simulink model "readProximity_sol"  (R2024a)
settings: Solver=FixedStepAuto  StartTime=0.0  StopTime=inf  RelTol=1e-9  EnableMultiTasking=on
undefined symbols (not defined in the file or in its folder): ln
libraries: arduinolib x2
settings Model: ExtModeTrigDuration=2  Creator=twallema  LastModifiedBy=twallema
settings SolverCC: AlgebraicLoopSolver=TrustRegion
settings OptimizationCC: EnhancedBackFolding=on  PassReuseOutputArgsThreshold=0  MaxStackSize=64  OptimizeBlockOrder=speed  DifferentSizesBufferReuse=on  OptimizationCustomize=off
settings DebuggingCC: ParameterTunabilityLossMsg=error  UnconnectedInputMsg=warning  UnconnectedOutputMsg=warning  UnconnectedLineMsg=warning
settings HardwareCC: ProdBitPerInt=16  ProdBitPerPointer=16  ProdBitPerSizeT=16  ProdBitPerPtrDiffT=16  ProdLargestAtomicFloat=None  ProdWordSize=8  ProdHWDeviceType=Atmel->AVR  UseEmbeddedCoderFeatures=off  UseSimulinkCoderFeatures=off
settings ModelReferenceCC: EnableRefExpFcnMdlSchedulingChecks=on
settings SFSimCC: MATLABDynamicMemAlloc=off  CustomCodeUndefinedFunction=UseInterfaceOnly
settings RTWCC: Description=Embedded Coder  SystemTargetFile=ert.tlc  HardwareBoard=Arduino Uno  TemplateMakefile=ert_default_tmf  GenerateReport=on  Toolchain=Arduino AVR  BuildConfiguration=Faster Runs  LaunchReport=on  GPUComputeCapability=3.5  DLArmComputeVersion=19.05
settings CodeAppCC: ForceParamTrailComments=on  OperatorAnnotations=on
settings ERTTargetCC: ERTCustomFileBanners=off  SupportContinuousTime=on  SupportNonInlinedSFcns=on  RemoveResetFunc=off  SupportVariableSizeSignals=on  ModelStepFunctionPrototypeControlCompliant=off  ExtModeStaticAllocSize=250

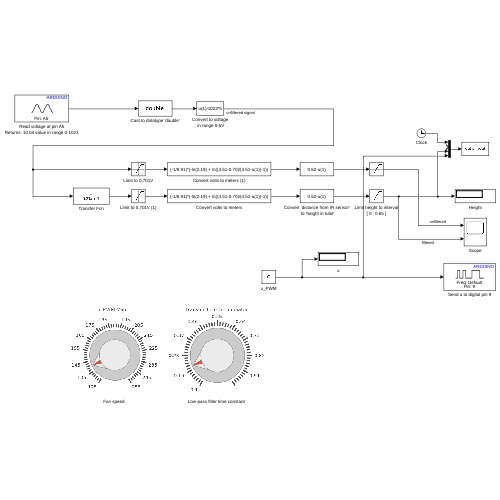
[thumbnail: Simulink's stored preview of the top-level diagram]
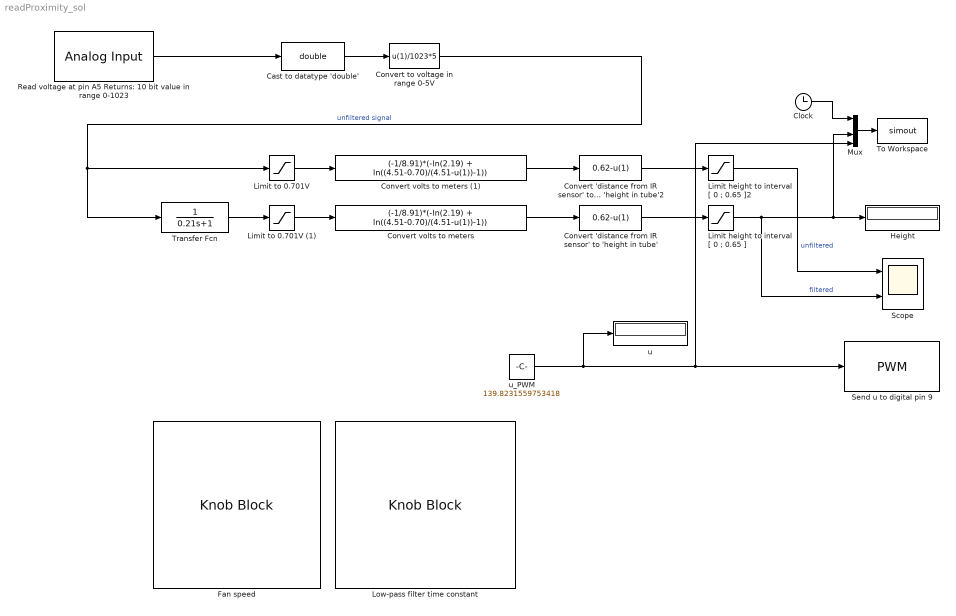
== system readProximity_sol ==
  Cast to datatype 'double' : DataTypeConversion  OutDataTypeStr=double  SaturateOnIntegerOverflow=off  RndMeth=Floor
  Clock : Clock
  Convert 'distance from IR sensor' to 'height in tube' : Fcn  Expr=0.62-u(1)
  Convert 'distance from IR sensor' to 'height in tube'2 : Fcn  Expr=0.62-u(1)
  Convert to voltage in range 0-5V : Fcn  Expr=u(1)/1023*5
  Convert volts to meters : Fcn  Expr=(-1/8.91)*(-ln(2.19) + ln((4.51-0.70)/(4.51-u(1))-1))
  Convert volts to meters (1) : Fcn  Expr=(-1/8.91)*(-ln(2.19) + ln((4.51-0.70)/(4.51-u(1))-1))
  Fan speed : KnobBlock  ScaleMin=125  ScaleMax=255
  Height : Display
  Limit height to interval [ 0 ; 0.65 ] : Saturate  UpperLimit=0.65  LowerLimit=0
  Limit height to interval [ 0 ; 0.65 ]2 : Saturate  UpperLimit=0.65  LowerLimit=0
  Limit to 0.701V : Saturate  UpperLimit=inf  LowerLimit=0.701
  Limit to 0.701V (1) : Saturate  UpperLimit=inf  LowerLimit=0.701
  Low-pass filter time constant : KnobBlock  ScaleMin=0.1  ScaleMax=1
  Mux : Mux
  Read voltage at pin A5 Returns: 10 bit value in range 0-1023 : arduinolib/Analog Input  pinNumber=5  ReadResultsOnly=off  ConversionTriggerSource=Software  ExternalTriggerType=uint32(0)  OutputDataType=uint16  EnableConversionCompleteNotify=off  EnableOuputStatus=off  SampleTime=-1  blockPlatform=arduino
  Scope : Scope  NumInputPorts=2
  Send u to digital pin 9 : arduinolib/PWM  pinNumber=9  frequencyType=Default  desiredFrequency=490.2  achievableFrequency=490.2
  To Workspace : ToWorkspace  VariableName=simout  SampleTime=-1
  Transfer Fcn : TransferFcn  Denominator=[0.21,1]
  u : Display
  u_PWM : Constant  Value=139.8231559753418
  wires:
  Read voltage at pin A5 Returns: 10 bit value in range 0-1023/1 -> Cast to datatype 'double'/1
  Cast to datatype 'double'/1 -> Convert to voltage in range 0-5V/1
  u_PWM/1 -> Mux/4, Send u to digital pin 9/1, u/1
  Mux/1 -> To Workspace/1
  Clock/1 -> Mux/1
  Convert 'distance from IR sensor' to 'height in tube'/1 -> Limit height to interval [ 0 ; 0.65 ]/1
  Limit height to interval [ 0 ; 0.65 ]2/1 -> Scope/1  "unfiltered"
  Limit height to interval [ 0 ; 0.65 ]/1 -> Scope/2, Mux/3, Height/1  "filtered"
  Convert volts to meters (1)/1 -> Convert 'distance from IR sensor' to 'height in tube'2/1
  Convert 'distance from IR sensor' to 'height in tube'2/1 -> Limit height to interval [ 0 ; 0.65 ]2/1
  Convert volts to meters/1 -> Convert 'distance from IR sensor' to 'height in tube'/1
  Limit to 0.701V/1 -> Convert volts to meters (1)/1
  Transfer Fcn/1 -> Limit to 0.701V (1)/1
  Limit to 0.701V (1)/1 -> Convert volts to meters/1
  Convert to voltage in range 0-5V/1 -> Transfer Fcn/1, Limit to 0.701V/1  "unfiltered signal"
